simulink model "simulation"  (R2021a)
settings: Solver=ode4  StartTime=0.0  StopTime=inf  FixedStep=0.002  RelTol=1e-3  EnableMultiTasking=on
libraries: simulink_extras x4, quarc_library x2
settings Model: ExtModeTrigDuration=10000  Creator=ADMIN  LastModifiedBy=ADMIN
settings SolverCC: AlgebraicLoopSolver=TrustRegion  PositivePriorityOrder=on
settings DataIOCC: ReturnWorkspaceOutputs=off
settings DebuggingCC: SFMachineParentedDataDiag=warning  ArithmeticOperatorsInVariantConditions=warning
settings SFSimCC: SimUseLocalCustomCode=off  CustomCodeUndefinedFunction=UseInterfaceOnly
settings RTWCC: Description=QUARC Win64 Target Using Toolchain  SystemTargetFile=quarc_win64.tlc  TemplateMakefile=quarc_default_tmf  RTWUseLocalCustomCode=off  Toolchain=QUARC win64 | nmake (64-bit Windows)  BuildConfiguration=Faster Runs
settings CodeAppCC: StateflowObjectComments=on
settings STFCustomTargetCC: TargetLangStandard=C99 (ISO)  ConcurrentExecutionCompliant=on  SystemTargetFile=quarc_win64.tlc
settings GRTTargetCC: ParMdlRefBuildCompliant=off  CompOptLevelCompliant=off  CombineOutputUpdateFcns=off  MatFileLogging=off  CPPClassGenCompliant=off  GRTInterface=on  ExtMode=on  ExtModeMexFile=quarc_comm
settings ConfigComp: CovMetricSettings=dswe

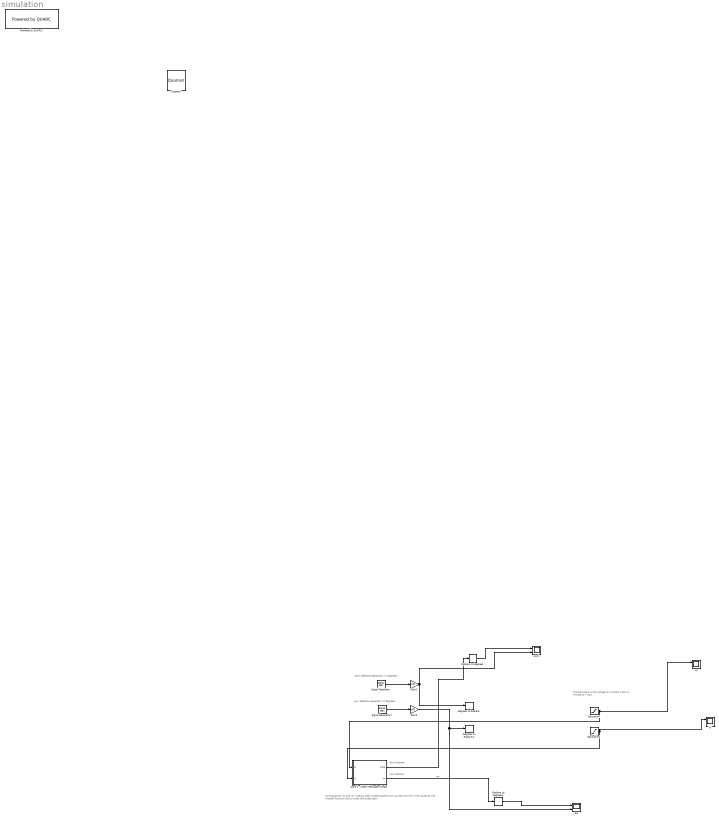
== system simulation ==
  note: pitch(radians)
  note: yaw(radians)
  note: pitch reference generator (in degrees)
  note: yaw reference generator (in degrees)
  note: The PID output is the voltage to 2 motors which is limited to +-24V
  note: Use equations (3) and (4) in aero2_2dof_modelling.pdf which you derive to fill in the values for the transfer function blocks inside this subsystem
  Aero 2 - 2 DOF Helicopter Model : Subsystem
  Degrees to Radians : simulink_extras/Transformations/Degrees to Radians
  Degrees to Radians1 : simulink_extras/Transformations/Degrees to Radians
  Gain2 : Gain  Gain=20
  Gain3 : Gain  Gain=45
  Powered by QUARC : quarc_library/Logos/Powered by QUARC
  Quanser : quarc_library/Logos/Quanser
  Radians to Degrees : simulink_extras/Transformations/Radians to Degrees
  Radians to Degrees1 : simulink_extras/Transformations/Radians to Degrees
  Saturation : Saturate  UpperLimit=24  LowerLimit=-24
  Saturation1 : Saturate  UpperLimit=24  LowerLimit=-24
  Signal Generator : SignalGenerator  WaveForm=square  Frequency=0.05
  Signal Generator1 : SignalGenerator  WaveForm=square  Frequency=0.04
  pitch : Scope  NumInputPorts=2
      settings: Description=pitch
  vp : Scope  NumInputPorts=2
      settings: Description=pitch
  vy : Scope  NumInputPorts=2
  yaw : Scope  NumInputPorts=2
  wires:
  Aero 2 - 2 DOF Helicopter Model/2(psi) -> Radians to Degrees1/1  "psi"
  Gain2/1 -> Degrees to Radians/1, pitch/2
  Signal Generator/1 -> Gain2/1
  Radians to Degrees/1 -> pitch/1
  Radians to Degrees1/1 -> yaw/1
  Saturation1/1 -> Aero 2 - 2 DOF Helicopter Model/2(Vy), vy/1
  Saturation/1 -> Aero 2 - 2 DOF Helicopter Model/1(Vp), vp/1
  Signal Generator1/1 -> Gain3/1
  Gain3/1 -> yaw/2, Degrees to Radians1/1
  Aero 2 - 2 DOF Helicopter Model/1(theta) -> Radians to Degrees/1

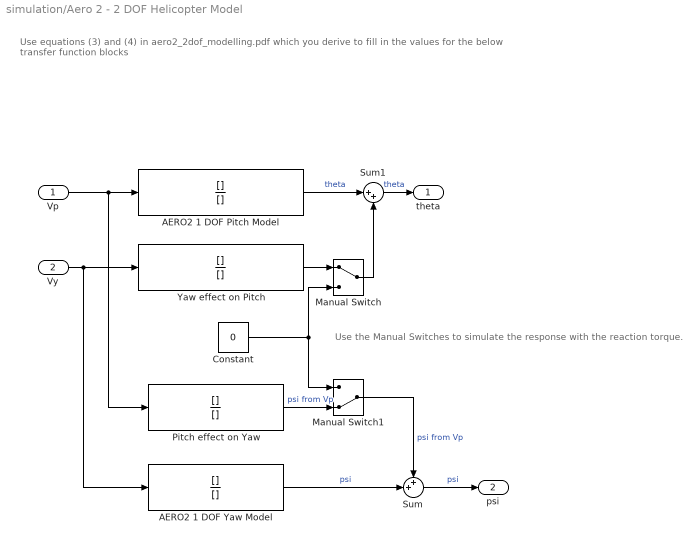
== system simulation/Aero 2 - 2 DOF Helicopter Model ==
  note: Use the Manual Switches to simulate the response with the reaction torque.
  note: Use equations (3) and (4) in aero2_2dof_modelling.pdf which you derive to fill in the values for the below transfer function blocks
  Vp : Inport
  Vy : Inport  Port=2
  "AERO2 1 DOF Pitch Model " : TransferFcn  Numerator=[]  Denominator=[]
  AERO2 1 DOF Yaw Model : TransferFcn  Numerator=[]  Denominator=[]
  Constant : Constant  Value=0
  Manual Switch : ManualSwitch
  Manual Switch1 : ManualSwitch  CurrentSetting=0
  Pitch effect on Yaw : TransferFcn  Numerator=[]  Denominator=[]
  Sum : Sum  Inputs=++|
  Sum1 : Sum  Inputs=|++
  Yaw effect on Pitch : TransferFcn  Numerator=[]  Denominator=[]
  theta : Outport
  psi : Outport  Port=2
  wires:
  "AERO2 1 DOF Pitch Model "/1 -> Sum1/1  "theta"
  Pitch effect on Yaw/1 -> Manual Switch1/2  "psi from Vp"
  Constant/1 -> Manual Switch1/1, Manual Switch/2
  Manual Switch/1 -> Sum1/2
  Yaw effect on Pitch/1 -> Manual Switch/1
  Vy/1 -> AERO2 1 DOF Yaw Model/1, Yaw effect on Pitch/1
  Vp/1 -> Pitch effect on Yaw/1, "AERO2 1 DOF Pitch Model "/1
  Sum1/1 -> theta/1  "theta"
  Manual Switch1/1 -> Sum/1  "psi from Vp"
  Sum/1 -> psi/1  "psi"
  AERO2 1 DOF Yaw Model/1 -> Sum/2  "psi"
